simulink model "hybrid_control"  (R2016a)
settings: Solver=VariableStepAuto  StartTime=0.0  StopTime=0.5  RelTol=1e-5
values from neighbouring files (symbols this model uses):
  Ts = 0.5e-3    (= 0.0005)    [generate_lookup_table.m]    (also in generator_script.m)
  ws_lt = -10000 : 1000 :10000    [generate_lookup_table.m]
undefined symbols (not defined in the file or in its folder): Ad_lt, Bd_lt, Cd_lt, DiscIntNeverNeededParam, Kdi_lt, Kdo_lt
settings Model: Creator=manuel  LastModifiedBy=manuel

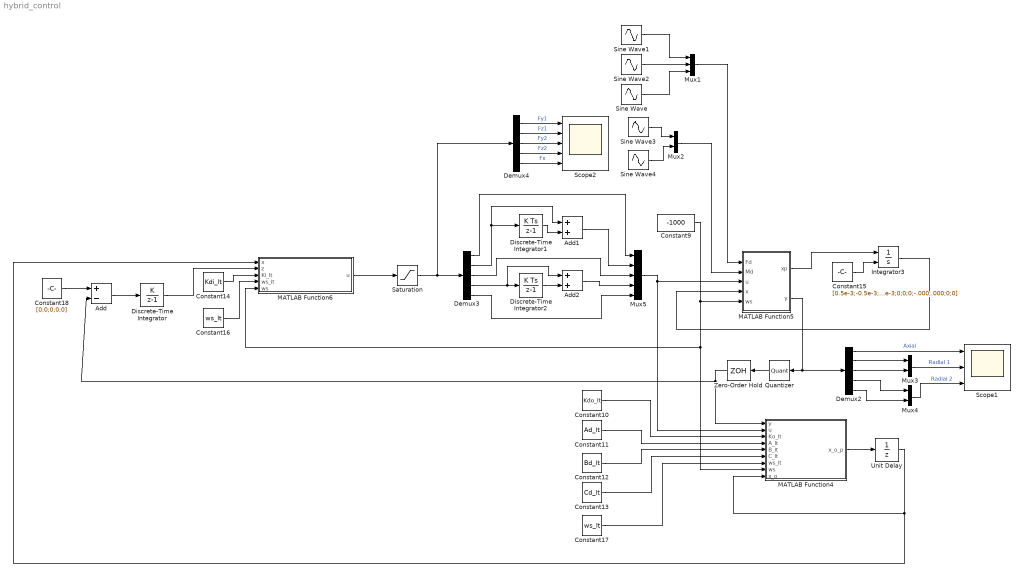
== system hybrid_control ==
  Add : Sum  Inputs=+-
  Add1 : Sum
  Add2 : Sum
  Constant10 : Constant  Value=Kdo_lt  VectorParams1D=off
  Constant11 : Constant  Value=Ad_lt  VectorParams1D=off
  Constant12 : Constant  Value=Bd_lt  VectorParams1D=off
  Constant13 : Constant  Value=Cd_lt  VectorParams1D=off
  Constant14 : Constant  Value=Kdi_lt  VectorParams1D=off
  Constant15 : Constant  Value=[0.5e-3;-0.5e-3;1e-3;0;0;0;-.000;.000;0;0]
  Constant16 : Constant  Value=ws_lt  VectorParams1D=off
  Constant17 : Constant  Value=ws_lt  VectorParams1D=off
  Constant18 : Constant  Value=[0;0;0;0;0]
  Constant9 : Constant  Value=-1000  VectorParams1D=off
  Demux2 : Demux  Outputs=5
  Demux3 : Demux  Outputs=5
  Demux4 : Demux  Outputs=5
  Discrete-Time Integrator : DiscreteIntegrator  IntegratorMethod=Accumulation: Forward Euler  InitialConditionSetting=State (most efficient)  SampleTime=-1  ICPrevOutput=DiscIntNeverNeededParam  ICPrevScaledInput=DiscIntNeverNeededParam
  Discrete-Time Integrator1 : DiscreteIntegrator  gainval=Kh  InitialConditionSetting=State (most efficient)  SampleTime=-1  ICPrevOutput=DiscIntNeverNeededParam  ICPrevScaledInput=DiscIntNeverNeededParam
  Discrete-Time Integrator2 : DiscreteIntegrator  gainval=Kh  InitialConditionSetting=State (most efficient)  SampleTime=-1  ICPrevOutput=DiscIntNeverNeededParam  ICPrevScaledInput=DiscIntNeverNeededParam
  Integrator3 : Integrator  InitialConditionSource=external
  MATLAB Function4 : MATLAB Function  TreatAsAtomicUnit=on
  MATLAB Function5 : MATLAB Function  TreatAsAtomicUnit=on
  MATLAB Function6 : MATLAB Function  TreatAsAtomicUnit=on
  Mux1 : Mux  Inputs=3
  Mux2 : Mux  Inputs=2
  Mux3 : Mux  Inputs=2
  Mux4 : Mux  Inputs=2
  Mux5 : Mux  Inputs=5
  Quantizer : Quantizer  QuantizationInterval=(2e-3)/256
  Saturation : Saturate  UpperLimit=10  LowerLimit=-10
  Scope1 : Scope  NumInputPorts=3
  Scope2 : Scope  NumInputPorts=5
  Sine Wave : Sin  Amplitude=3  Bias=10  Frequency=100*2*pi  SampleTime=0
  Sine Wave1 : Sin  Frequency=50*2*pi  SampleTime=0
  Sine Wave2 : Sin  Frequency=100*2*pi  SampleTime=0
  Sine Wave3 : Sin  Amplitude=0  Frequency=600*2*pi  SampleTime=0
  Sine Wave4 : Sin  Amplitude=0  Frequency=300*2*pi  SampleTime=0
  Unit Delay : UnitDelay  InitialCondition=[0;0;0;0;0;0;0;0;0;0]  SampleTime=-1
  Zero-Order Hold : ZeroOrderHold  SampleTime=Ts
  wires:
  ? -> ?
  Constant15/1 -> Integrator3/2
  Integrator3/1 -> MATLAB Function5/4(x)
  Constant14/1 -> MATLAB Function6/3(Ki_lt)
  MATLAB Function5/1(xp) -> Integrator3/1
  MATLAB Function4/1(x_o_p) -> Unit Delay/1
  Constant10/1 -> MATLAB Function4/3(Ko_lt)
  Constant11/1 -> MATLAB Function4/4(A_lt)
  Constant12/1 -> MATLAB Function4/5(B_lt)
  Constant13/1 -> MATLAB Function4/6(C_lt)
  Constant9/1 -> MATLAB Function6/5(ws), MATLAB Function4/8(ws), MATLAB Function5/5(ws)
  Constant16/1 -> MATLAB Function6/4(ws_lt)
  Constant17/1 -> MATLAB Function4/7(ws_lt)
  Demux2/2 -> Mux3/1
  Demux2/3 -> Mux3/2
  Demux2/4 -> Mux4/1
  Demux2/5 -> Mux4/2
  MATLAB Function5/2(y) -> Demux2/1, Quantizer/1
  Mux3/1 -> Scope1/2  "Radial 1"
  Mux4/1 -> Scope1/3  "Radial 2"
  Constant18/1 -> Add/1
  Add/1 -> Discrete-Time Integrator/1
  Discrete-Time Integrator/1 -> MATLAB Function6/2(z)
  Zero-Order Hold/1 -> Add/2, MATLAB Function4/1(y)
  Mux5/1 -> MATLAB Function4/2(u), MATLAB Function5/3(u)
  Discrete-Time Integrator1/1 -> Add1/2
  Discrete-Time Integrator2/1 -> Add2/2
  Demux4/1 -> Scope2/1  "Fy1"
  Demux4/2 -> Scope2/2  "Fz1"
  Demux4/3 -> Scope2/3  "Fy2"
  Demux4/4 -> Scope2/4  "Fz2"
  Demux4/5 -> Scope2/5  "Fx"
  Demux3/4 -> Add2/1, Discrete-Time Integrator2/1
  Add2/1 -> Mux5/4
  Add1/1 -> Mux5/2
  Demux3/2 -> Add1/1, Discrete-Time Integrator1/1
  Demux3/3 -> Mux5/3
  Demux3/1 -> Mux5/1
  Demux3/5 -> Mux5/5
  Demux2/1 -> Scope1/1  "Axial"
  Mux2/1 -> MATLAB Function5/2(Md)
  Mux1/1 -> MATLAB Function5/1(Fd)
  Saturation/1 -> Demux4/1, Demux3/1
  MATLAB Function6/1(u) -> Saturation/1
  Sine Wave3/1 -> Mux2/1
  Sine Wave4/1 -> Mux2/2
  Sine Wave2/1 -> Mux1/2
  Sine Wave/1 -> Mux1/3
  Sine Wave1/1 -> Mux1/1
  Quantizer/1 -> Zero-Order Hold/1
  Unit Delay/1 -> MATLAB Function4/9(x_o), MATLAB Function6/1(x)

== matlab function hybrid_control/MATLAB Function4 ==
  data: y input; u input; x_o_p output; Ko_lt input; A_lt input; B_lt input; C_lt input; ws_lt input; ws input; x_o input
function x_o_p = state_obsever(y,u,Ko_lt,A_lt,B_lt,C_lt,ws_lt,ws,x_o)
%#codegen
Ko = matrix_interpolation(ws_lt,Ko_lt,ws);
A = matrix_interpolation(ws_lt,A_lt,ws);
B = matrix_interpolation(ws_lt,B_lt,ws);
C = matrix_interpolation(ws_lt,C_lt,ws);

x_o_p = A*x_o + B*u + Ko*(y-C*x_o);

== matlab function hybrid_control/MATLAB Function5 ==
  data: Fd input; Md input; u input; x input; xp output; y output; ws input
function [xp,y] = fcn(Fd,Md,u,x,ws)

Fd_x = Fd(1);
Fd_y = Fd(2);
Fd_z = Fd(3);
Md_y = Md(1);
Md_z = Md(2);

[xp,y] = hmb_non_linear_model(x,u,ws,Fd_x,Fd_y,Fd_z,Md_y,Md_z);

end

== matlab function hybrid_control/MATLAB Function6 ==
  data: x input; z input; Ki_lt input; ws_lt input; u output; ws input
function u  = feedback_controller(x,z,Ki_lt,ws_lt,ws)
%#codegen
ki = matrix_interpolation(ws_lt,Ki_lt,ws);

xi = [x;z];

u = -ki*xi;
